simulink model "Copy_of_J3"  (R2019b)
settings: Solver=VariableStepAuto  StartTime=0.0  StopTime=10.0  RelTol=1e-3
settings Model: Creator=Inspiron  LastModifiedBy=Inspiron

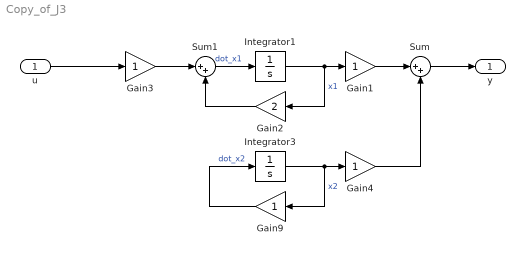
== system Copy_of_J3 ==
  u : Inport
  Gain{1,3..4,9} (4 alike) : Gain
  Gain2 : Gain  Gain=2
  Integrator1 : Integrator
  Integrator3 : Integrator
  Sum : Sum  Inputs=|++
  Sum1 : Sum  Inputs=|++
  y : Outport
  wires:
  u/1 -> Gain3/1
  Sum/1 -> y/1
  Sum1/1 -> Integrator1/1  "dot_x1"
  Integrator1/1 -> Gain1/1, Gain2/1  "x1"
  Gain2/1 -> Sum1/2
  Gain9/1 -> Integrator3/1  "dot_x2"
  Integrator3/1 -> Gain4/1, Gain9/1  "x2"
  Gain3/1 -> Sum1/1
  Gain1/1 -> Sum/1
  Gain4/1 -> Sum/2
